simulink model "relative_dist_and_velocity_plausibility_AEB"  (R2021a)
settings: Solver=VariableStepAuto  StartTime=0.0  StopTime=10.0  RelTol=1e-3
settings Model: Creator=uidk9388  LastModifiedBy=uidk9388

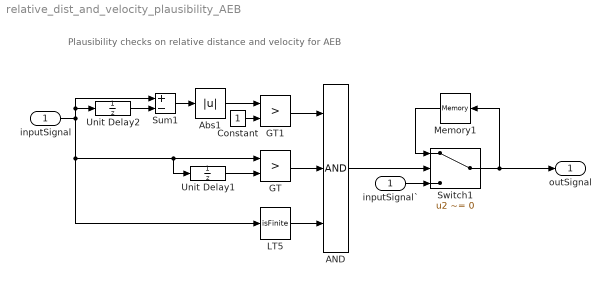
== system relative_dist_and_velocity_plausibility_AEB ==
  note: Plausibility checks on relative distance and velocity for AEB
  inputSignal : Inport
  AND : Logic  Inputs=3  IconShape=distinctive  AllPortsSameDT=off  OutDataTypeStr=boolean
      mask Display: disp('AND')
  Abs1 : Abs
  Constant : Constant
  GT : RelationalOperator  Operator=>  OutDataTypeStr=boolean  RndMeth=Simplest
  GT1 : RelationalOperator  Operator=>  OutDataTypeStr=boolean  RndMeth=Simplest
  LT5 : RelationalOperator  Operator=isFinite  OutDataTypeStr=boolean  RndMeth=Simplest
  Memory1 : Memory
  Sum1 : Sum  Inputs=+-
  Switch1 : Switch  Criteria=u2 ~= 0  Threshold=0.4
  Unit Delay1 : UnitDelay  SampleTime=-1  HasFrameUpgradeWarning=on
  Unit Delay2 : UnitDelay  SampleTime=-1  HasFrameUpgradeWarning=on
  inputSignal` : InportShadow
  outSignal : Outport
  wires:
  GT/1 -> AND/2
  Switch1/1 -> Memory1/1, outSignal/1
  inputSignal/1 -> LT5/1, Unit Delay1/1, GT/1, Sum1/1, Unit Delay2/1
  LT5/1 -> AND/3
  Constant/1 -> GT1/2
  inputSignal`/1 -> Switch1/3
  GT1/1 -> AND/1
  Sum1/1 -> Abs1/1
  AND/1 -> Switch1/2
  Unit Delay1/1 -> GT/2
  Abs1/1 -> GT1/1
  Memory1/1 -> Switch1/1
  Unit Delay2/1 -> Sum1/2
